simulink model "pendulumSimPID"  (R2024b)
settings: Solver=FixedStepAuto  StartTime=0.0  StopTime=4  FixedStep=0.001  MaxStep=0.005  RelTol=1e-3
settings Model: Creator=mattf  LastModifiedBy=nicholas

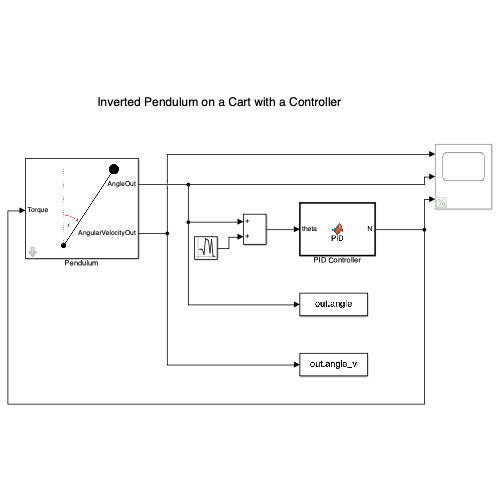
[thumbnail: Simulink's stored preview of the top-level diagram]
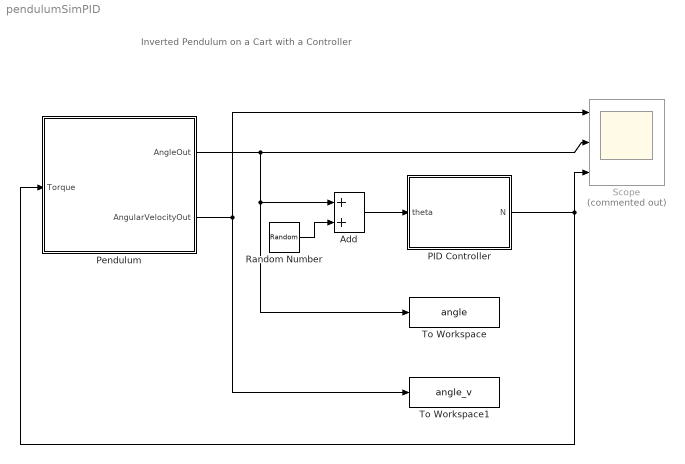
== system pendulumSimPID ==
  note: Inverted Pendulum on a Cart with a Controller
  Add : Sum
  PID Controller : MATLAB Function  TreatAsAtomicUnit=on
  Pendulum : Subsystem  mask{m=0.2, l=0.3/2, g=9.8, init=pi/6}
      mask prompts: m "Pend Mass (kg):"; l "COM Distance (m):"; g "Acc due to Gravity (g):"; init "Initial Angle (rad):"
      mask Display: image('pen img.png');
  Random Number : RandomNumber  SampleTime=0.001
  Scope : Scope  Commented=on  NumInputPorts=3
  To Workspace : ToWorkspace  VariableName=angle  SampleTime=-1
  To Workspace1 : ToWorkspace  VariableName=angle_v  SampleTime=-1
  wires:
  Pendulum/2(AngularVelocityOut) -> To Workspace1/1, Scope/1
  Pendulum/1(AngleOut) -> Add/1, To Workspace/1, Scope/2
  Random Number/1 -> Add/2
  Add/1 -> PID Controller/1(theta)
  PID Controller/1(N) -> Scope/3, Pendulum/1(Torque)

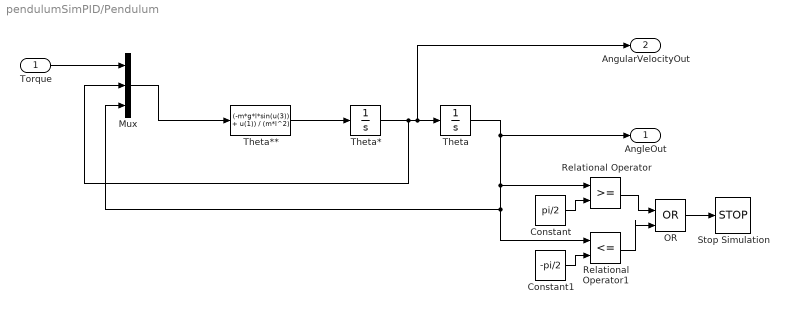
== system pendulumSimPID/Pendulum ==
  Torque : Inport
  Constant : Constant  Value=pi/2
  Constant1 : Constant  Value=-pi/2
  Mux : Mux  Inputs=3
  OR : Logic  Operator=OR  IconShape=distinctive  AllPortsSameDT=off  OutDataTypeStr=boolean
  Relational Operator : RelationalOperator  OutDataTypeStr=boolean  RndMeth=Simplest  InputSameDT=off
  Relational Operator1 : RelationalOperator  Operator=<=  OutDataTypeStr=boolean  RndMeth=Simplest  InputSameDT=off
  Stop Simulation : Stop
  Theta : Integrator  InitialCondition=init
  Theta* : Integrator
  Theta** : Fcn  Expr=(-m*g*l*sin(u(3)) + u(1)) / (m*l^2)
  AngleOut : Outport
  AngularVelocityOut : Outport  Port=2
  wires:
  Constant1/1 -> Relational Operator1/2
  Theta**/1 -> Theta*/1
  Theta/1 -> AngleOut/1, Relational Operator1/1, Mux/3, Relational Operator/1
  OR/1 -> Stop Simulation/1
  Theta*/1 -> Mux/2, AngularVelocityOut/1, Theta/1
  Torque/1 -> Mux/1
  Relational Operator/1 -> OR/1
  Relational Operator1/1 -> OR/2
  Constant/1 -> Relational Operator/2
  Mux/1 -> Theta**/1

== matlab function pendulumSimPID/PID Controller ==
  settings: updateMethod=DISCRETE
  data: N output; theta input
function N = PID(theta)

    % call extrinsic python function
    coder.extrinsic('py.PIDControllerPendulum.controller_call');

    % Call Python function and return result
    N = coder.nullcopy(zeros(1,1)); % no clue why, but this is need.
    N = double(py.PIDControllerPendulum.controller_call(theta));
    end
